simulink model "test"  (R2022b)
settings: Solver=VariableStepAuto  StartTime=0.0  StopTime=10.0  RelTol=1e-3
settings Model: Creator=anton  LastModifiedBy=anton
settings DataIOCC: ExternalInput=data  LoadExternalInput=on

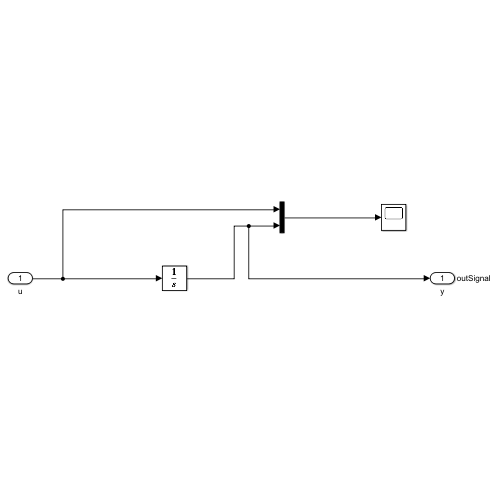
[thumbnail: Simulink's stored preview of the top-level diagram]
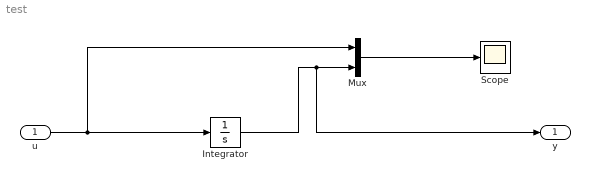
== system test ==
  u : Inport  PortDimensions=1
  Integrator : Integrator
  Mux : Mux  Inputs=2
  Scope : Scope
  y : Outport  SignalName=outSignal
  wires:
  u/1 -> Mux/1, Integrator/1
  Mux/1 -> Scope/1
  Integrator/1 -> y/1, Mux/2
